simulink model "Q7"  (R2020b)
settings: Solver=VariableStepAuto  StartTime=0.0  StopTime=10.0  RelTol=1e-3
settings Model: Creator=HP  LastModifiedBy=HP

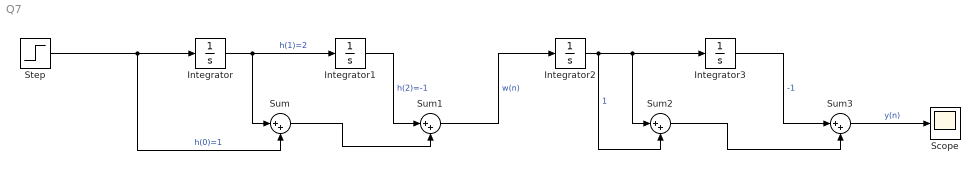
== system Q7 ==
  Integrator{,1..3} (4 alike) : Integrator
  Scope : Scope
  Step : Step  SampleTime=0
  Sum{,1..3} (4 alike) : Sum  Inputs=|++
  wires:
  Integrator/1 -> Sum/1, Integrator1/1  "h(1)=2"
  Step/1 -> Sum/2, Integrator/1  "h(0)=1"
  Integrator1/1 -> Sum1/1  "h(2)=-1"
  Integrator3/1 -> Sum3/1  "-1"
  Integrator2/1 -> Sum2/2, Sum2/1, Integrator3/1  "1"
  Sum1/1 -> Integrator2/1  "w(n)"
  Sum/1 -> Sum1/2
  Sum2/1 -> Sum3/2
  Sum3/1 -> Scope/1  "y(n)"
